simulink model "loopback_sinewave_withtout_PlutoSDR"  (R2021a)
settings: Solver=VariableStepAuto  StartTime=0.0  StopTime=0.01  RelTol=1e-3
InitFcn:
  | fs = 2e5;
  | frameSize = 1024;
libraries: dspsrcs4 x1, dsparch4 x1
settings Model: Creator=Byung-Jun Jang  LastModifiedBy=user
settings SolverCC: AlgebraicLoopSolver=TrustRegion
settings DataIOCC: ReturnWorkspaceOutputs=off
settings DebuggingCC: SFMachineParentedDataDiag=warning  ArithmeticOperatorsInVariantConditions=warning
settings SFSimCC: SimUseLocalCustomCode=off  CustomCodeUndefinedFunction=UseInterfaceOnly
settings RTWCC: RTWUseLocalCustomCode=off
settings CodeAppCC: StateflowObjectComments=on
settings SimscapeCC: SimscapeNormalizeSystem=off

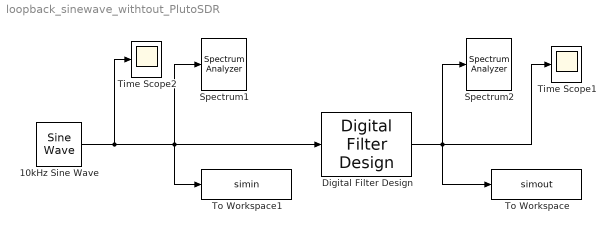
== system loopback_sinewave_withtout_PlutoSDR ==
  10kHz Sine Wave : dspsrcs4/Sine Wave  Amplitude=sqrt(1)  Frequency=10e3  Phase=0  SampleMode=Discrete  OutComplex=Complex  CompMethod=Trigonometric fcn  TableSize=Speed  SampleTime=1/fs  SamplesPerFrame=frameSize  ResetState=Restart at time zero  OutputFrames=off  dataType=single  wordLen=16  udDataType=sfix(16)  fracBitsMode=Best precision  numFracBits=15  OutDataTypeStr=single  LastOutDataTypeStr=single
  Digital Filter Design : dsparch4/Digital Filter Design  mwdsp_browser_bugfix_var=off
  Spectrum1 : SpectrumAnalyzer
  Spectrum2 : SpectrumAnalyzer
  Time Scope1 : Scope
  Time Scope2 : Scope
  To Workspace : ToWorkspace  VariableName=simout  SaveFormat=Timeseries  SampleTime=-1
  To Workspace1 : ToWorkspace  VariableName=simin  SaveFormat=Timeseries  SampleTime=-1
  wires:
  Digital Filter Design/1 -> Time Scope1/1, To Workspace/1, Spectrum2/1
  10kHz Sine Wave/1 -> Time Scope2/1, To Workspace1/1, Spectrum1/1, Digital Filter Design/1
